simulink model "malha_fechada_simu"  (R2018a)
settings: Solver=VariableStepAuto  StartTime=0.0  StopTime=7.0  RelTol=1e-3
values from neighbouring files (symbols this model uses):
  KIm = Pm*KPm    (= 0.751884057971)    [LineFollower.m]    (also in malha_fechada.m = 0.759312111233)
  Km = 460    [LineFollower.m]    (also in malha_aberta.m = 455.5; malha_fechada.m = 455.5)
  KPm = 4/(Km*ts_m)    (= 0.0579710144928)    [LineFollower.m]    (also in malha_fechada.m = 0.0585437248445)
  Pm = 12.97    [LineFollower.m]    (also in malha_aberta.m; malha_fechada.m)
  Ts = 1e-3    (= 0.001)    [LineFollower.m]    (also in Untitled.m; calculo_erros.m; ft_speedw.mat; malha_aberta.m)
libraries: simulink x1
settings Model: Creator=bruno  LastModifiedBy=bruno

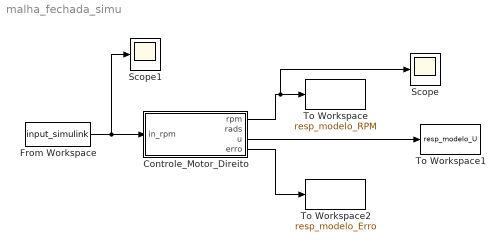
== system malha_fechada_simu ==
  Controle_Motor_Direito : Subsystem
  From Workspace : FromWorkspace  VariableName=input_simulink  SampleTime=Ts
  Scope : Scope
  Scope1 : Scope
  To Workspace : ToWorkspace  VariableName=resp_modelo_RPM  SampleTime=Ts
      settings: Save2DSignal=2-D array (concatenate along first dimension)
  To Workspace1 : ToWorkspace  VariableName=resp_modelo_U  SampleTime=Ts
      settings: Save2DSignal=2-D array (concatenate along first dimension)
  To Workspace2 : ToWorkspace  VariableName=resp_modelo_Erro  SampleTime=Ts
      settings: Save2DSignal=2-D array (concatenate along first dimension)
  wires:
  From Workspace/1 -> Scope1/1, Controle_Motor_Direito/1(in_rpm)
  Controle_Motor_Direito/1(rpm) -> Scope/1, To Workspace/1
  Controle_Motor_Direito/3(u) -> To Workspace1/1
  Controle_Motor_Direito/4(erro) -> To Workspace2/1

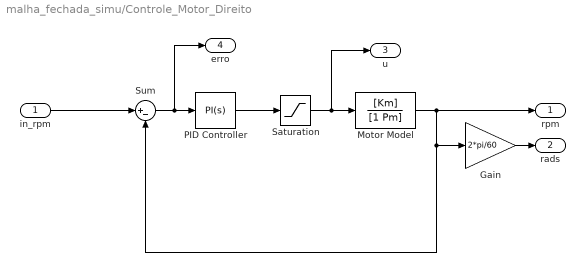
== system malha_fechada_simu/Controle_Motor_Direito ==
  in_rpm : Inport
  Gain : Gain  Gain=2*pi/60
  Motor Model : TransferFcn  Numerator=[Km]  Denominator=[1 Pm]
  PID Controller : simulink/Continuous/PID Controller  Controller=PI  TimeDomain=Continuous-time  SampleTime=-1  IntegratorMethod=Forward Euler  FilterMethod=Forward Euler  Form=Parallel  UseFilter=on  ControllerParametersSource=internal  P=KPm  I=KIm  D=0  N=0  InitialConditionSource=internal  InitialConditionForIntegrator=0  InitialConditionForFilter=0  ExternalReset=none  LimitOutput=off  UpperSaturationLimit=inf  LowerSaturationLimit=-inf  LinearizeAsGain=on  AntiWindupMode=none  Kb=1  TrackingMode=off  Kt=1  PParamMin=[]  PParamMax=[]  IParamMin=[]  IParamMax=[]  DParamMin=[]  DParamMax=[]  NParamMin=[]  NParamMax=[]  KbParamMin=[]  KbParamMax=[]  KtParamMin=[]  KtParamMax=[]  POutMin=[]  POutMax=[]  IOutMin=[]  IOutMax=[]  DOutMin=[]  DOutMax=[]  NOutMin=[]  NOutMax=[]  KbOutMin=[]  KbOutMax=[]  KtOutMin=[]  KtOutMax=[]  IntegratorOutMin=[]  IntegratorOutMax=[]  FilterOutMin=[]  FilterOutMax=[]  SumOutMin=[]  SumOutMax=[]  SumI1OutMin=[]  SumI1OutMax=[]  SumI2OutMin=[]  SumI2OutMax=[]  SumI3OutMin=[]  SumI3OutMax=[]  SumDOutMin=[]  SumDOutMax=[]  SaturationOutMin=[]  SaturationOutMax=[]  IntegratorContinuousStateAttributes=''  IntegratorStateMustResolveToSignalObject=off  IntegratorRTWStateStorageClass=Auto  FilterContinuousStateAttributes=''  FilterStateMustResolveToSignalObject=off  FilterRTWStateStorageClass=Auto  DifferentiatorICPrevScaledInput=0  DifferentiatorOutMin=[]  DifferentiatorOutMax=[]  FilterDiffOutCoefMin=[]  FilterDiffOutCoefMax=[]  SumDenOutMin=[]  SumDenOutMax=[]  SumNumOutMin=[]  SumNumOutMax=[]  ReciprocalOutMin=[]  ReciprocalOutMax=[]  DivideOutMin=[]  DivideOutMax=[]  TunerSelectOption=Transfer Function Based (PID Tuner App)
  Saturation : Saturate  UpperLimit=100  LowerLimit=-100
  Sum : Sum  Inputs=|+-
  rpm : Outport
  rads : Outport  Port=2
  u : Outport  Port=3
  erro : Outport  Port=4
  wires:
  PID Controller/1 -> Saturation/1
  Motor Model/1 -> rpm/1, Gain/1, Sum/2
  Saturation/1 -> u/1, Motor Model/1
  Sum/1 -> erro/1, PID Controller/1
  in_rpm/1 -> Sum/1
  Gain/1 -> rads/1
